simulink model "BehPlantHyperCook"  (R2026a)
settings: Solver=VariableStepAuto  StopTime=14400
undefined symbols (not defined in the file): HC_PackRate_bph, HC_QCRate_bph, HC_Resupply_bph, HC_StaticPower_kW
settings Model: DataDictionary=BehParamsHyperCook.sldd  Creator=sarah  LastModifiedBy=sarah

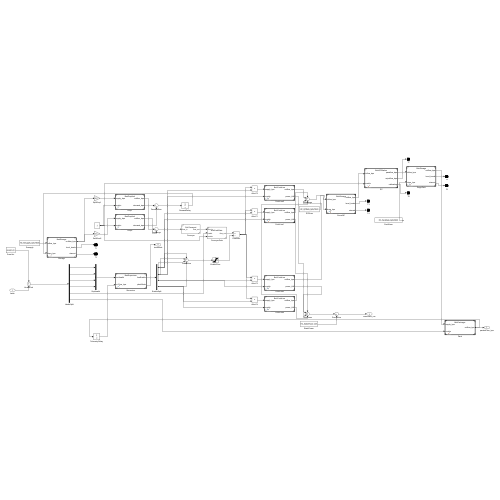
[thumbnail: Simulink's stored preview of the top-level diagram]
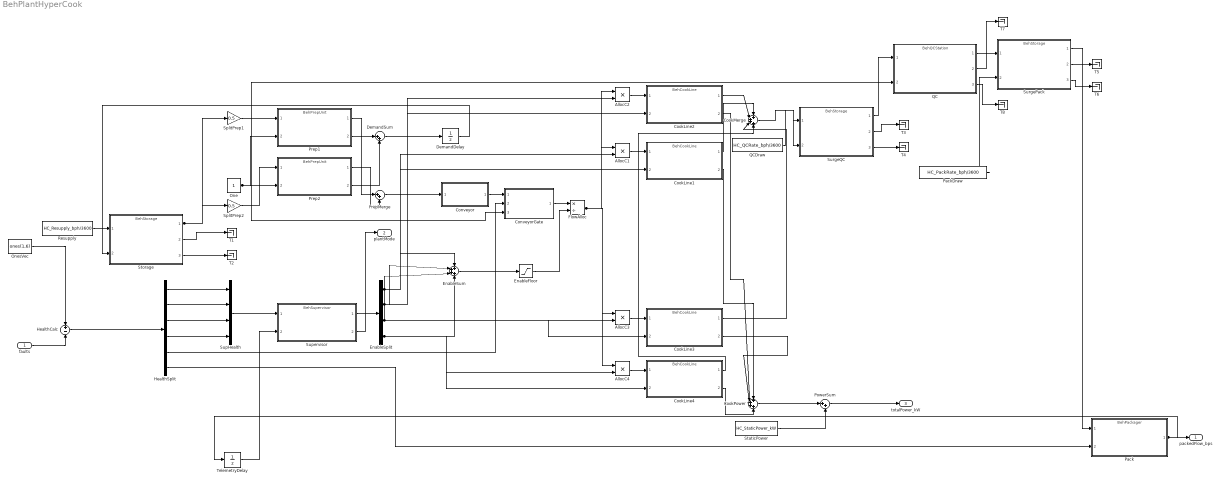
== system BehPlantHyperCook ==
  faults : Inport  PortDimensions=6
  AllocC{1..4} (4 alike) : Product
  Conveyor : Subsystem  ReferencedSubsystem=SubTransport
  ConveyorGate : Subsystem  ReferencedSubsystem=SubFaultGate
  CookLine{1..4} (4 alike) : ModelReference  ModelNameDialog=BehCookLine  UsingDefaultArgumentValue=0,0,0,0  SimulationMode=Normal  ModelReferenceVersion=1.4
  CookMerge : Sum  Inputs=++++
  CookPower : Sum  Inputs=++++
  DemandDelay : UnitDelay
  DemandSum : Sum  Inputs=|++
  EnableFloor : Saturate  UpperLimit=inf  LowerLimit=1
  EnableSplit : Demux
  EnableSum : Sum  Inputs=++++
  FlowAlloc : Product  Inputs=*/
  HealthCalc : Sum  Inputs=+-
  HealthSplit : Demux  Outputs=6
  One : Constant
  OnesVec : Constant  Value=ones(1,6)
  Pack : ModelReference  ModelNameDialog=BehPackager  UsingDefaultArgumentValue=0,0  SimulationMode=Normal  ModelReferenceVersion=1.4
  PackDraw : Constant  Value=HC_PackRate_bph/3600
  PowerSum : Sum  Inputs=|++
  Prep1 : ModelReference  ModelNameDialog=BehPrepUnit  UsingDefaultArgumentValue=0,0  SimulationMode=Normal  ModelReferenceVersion=1.4
  Prep2 : ModelReference  ModelNameDialog=BehPrepUnit  UsingDefaultArgumentValue=0,0  SimulationMode=Normal  ModelReferenceVersion=1.4
  PrepMerge : Sum  Inputs=|++
  QC : ModelReference  ModelNameDialog=BehQCStation  UsingDefaultArgumentValue=0,0,0,0  SimulationMode=Normal  ModelReferenceVersion=1.4
  QCDraw : Constant  Value=HC_QCRate_bph/3600
  Resupply : Constant  Value=HC_Resupply_bph/3600
  SplitPrep1 : Gain  Gain=0.5
  SplitPrep2 : Gain  Gain=0.5
  StaticPower : Constant  Value=HC_StaticPower_kW
  Storage : ModelReference  ModelNameDialog=BehStorage  UsingDefaultArgumentValue=0,0  SimulationMode=Normal  ModelReferenceVersion=1.3
  SupHealth : Mux
  Supervisor : ModelReference  ModelNameDialog=BehSupervisor  ParameterArgumentNames=NumLines  ParameterArgumentValues=HC_NumLines  UsingDefaultArgumentValue=0  SimulationMode=Normal  ModelReferenceVersion=1.6
  SurgePack : ModelReference  ModelNameDialog=BehStorage  UsingDefaultArgumentValue=0,0  SimulationMode=Normal  ModelReferenceVersion=1.3
  SurgeQC : ModelReference  ModelNameDialog=BehStorage  UsingDefaultArgumentValue=0,0  SimulationMode=Normal  ModelReferenceVersion=1.3
  T{1..8} (8 alike) : Terminator
  TelemetryDelay : UnitDelay
  packedFlow_bps : Outport
  plantMode : Outport  Port=2
  totalPower_kW : Outport  Port=3
  wires:
  ConveyorGate/1 -> FlowAlloc/1
  EnableSplit/1 -> EnableSum/1, AllocC1/2, CookLine1/2
  Prep1/2 -> DemandSum/1
  OnesVec/1 -> HealthCalc/1
  Storage/3 -> T2/1
  CookLine1/1 -> CookMerge/1
  PrepMerge/1 -> Conveyor/1
  Prep2/2 -> DemandSum/2
  Storage/2 -> T1/1
  SupHealth/1 -> Supervisor/1
  One/1 -> ConveyorGate/3, Prep2/2, Prep1/2, QC/2
  HealthSplit/2 -> SupHealth/2
  Storage/1 -> SplitPrep2/1, SplitPrep1/1
  CookLine2/1 -> CookMerge/2
  HealthCalc/1 -> HealthSplit/1
  EnableSplit/3 -> EnableSum/3, AllocC3/2, CookLine3/2
  faults/1 -> HealthCalc/2
  Resupply/1 -> Storage/1
  StaticPower/1 -> PowerSum/2
  HealthSplit/1 -> SupHealth/1
  SurgePack/2 -> T5/1
  DemandDelay/1 -> Storage/2
  HealthSplit/3 -> SupHealth/3
  HealthSplit/4 -> SupHealth/4
  HealthSplit/5 -> ConveyorGate/2
  CookLine4/1 -> CookMerge/4
  HealthSplit/6 -> Pack/2
  SplitPrep1/1 -> Prep1/1
  SplitPrep2/1 -> Prep2/1
  TelemetryDelay/1 -> Supervisor/2
  PowerSum/1 -> totalPower_kW/1
  Prep1/1 -> PrepMerge/1
  CookLine1/2 -> CookPower/1
  Prep2/1 -> PrepMerge/2
  Supervisor/1 -> EnableSplit/1
  SurgePack/1 -> Pack/1
  Supervisor/2 -> plantMode/1
  DemandSum/1 -> DemandDelay/1
  EnableSplit/2 -> AllocC2/2, EnableSum/2, CookLine2/2
  AllocC4/1 -> CookLine4/1
  EnableSplit/4 -> EnableSum/4, CookLine4/2, AllocC4/2
  Conveyor/1 -> ConveyorGate/1
  CookLine2/2 -> CookPower/2
  EnableSum/1 -> EnableFloor/1
  EnableFloor/1 -> FlowAlloc/2
  PackDraw/1 -> SurgePack/2
  FlowAlloc/1 -> AllocC3/1, AllocC4/1, AllocC2/1, AllocC1/1
  QCDraw/1 -> SurgeQC/2
  AllocC2/1 -> CookLine2/1
  AllocC1/1 -> CookLine1/1
  AllocC3/1 -> CookLine3/1
  CookLine3/1 -> CookMerge/3
  CookLine3/2 -> CookPower/3
  SurgePack/3 -> T6/1
  CookLine4/2 -> CookPower/4
  SurgeQC/2 -> T3/1
  CookMerge/1 -> SurgeQC/1
  CookPower/1 -> PowerSum/1
  SurgeQC/1 -> QC/1
  SurgeQC/3 -> T4/1
  QC/1 -> SurgePack/1
  QC/2 -> T7/1
  QC/3 -> T8/1
  Pack/1 -> TelemetryDelay/1, packedFlow_bps/1
